simulink model "Plant"  (R2021a)
settings: Solver=VariableStepAuto  StartTime=0.0  StopTime=10.0  RelTol=1e-3
values from neighbouring files (symbols this model uses):
  I = [Jx Jxy Jxz ... (first row only)    [init.m]
  m = 1.5    [init.m]
  pos_ref = [ pos_refx' pos_refy' pos_refz' ]    [trajplann3.m]
  t_ref = []    [trajplann3.m]
  vel_ref = [ vel_refx, vel_refy, vel_refz ]    [trajplann3.m]
undefined symbols (not defined in the file or in its folder): psi, psi_dot
libraries: simulink x2
settings Model: Creator=iris  LastModifiedBy=iris

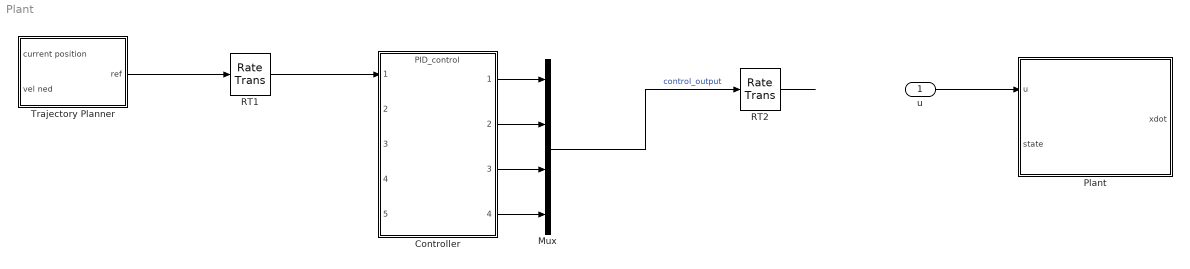
== system Plant ==
  u : Inport
  Controller : ModelReference  ModelNameDialog=PID_control  SimulationMode=Normal  ModelReferenceVersion=4.0
  Mux : Mux
  Plant : Subsystem
  RT1 : RateTransition  OutPortSampleTimeOpt=Inherit  OutPortSampleTime=0.01
  RT2 : RateTransition  OutPortSampleTimeOpt=Inherit  OutPortSampleTime=0.001
  Trajectory Planner : Subsystem
  wires:
  Controller/1 -> Mux/1
  Controller/2 -> Mux/2
  Controller/3 -> Mux/3
  Controller/4 -> Mux/4
  Trajectory Planner/1(ref) -> RT1/1
  RT1/1 -> Controller/1
  u/1 -> Plant/1(u)
  Mux/1 -> RT2/1  "control_output"
  RT2/1 -> ?

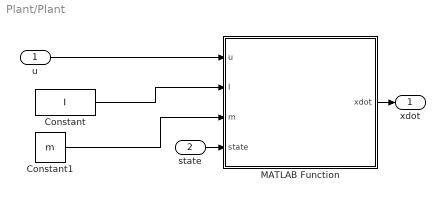
== system Plant/Plant ==
  u : Inport
  state : Inport  Port=2
  Constant : Constant  Value=I
  Constant1 : Constant  Value=m
  MATLAB Function : MATLAB Function  TreatAsAtomicUnit=on
  xdot : Outport
  wires:
  u/1 -> MATLAB Function/1(u)
  Constant1/1 -> MATLAB Function/3(m)
  MATLAB Function/1(xdot) -> xdot/1
  Constant/1 -> MATLAB Function/2(I)
  state/1 -> MATLAB Function/4(state)

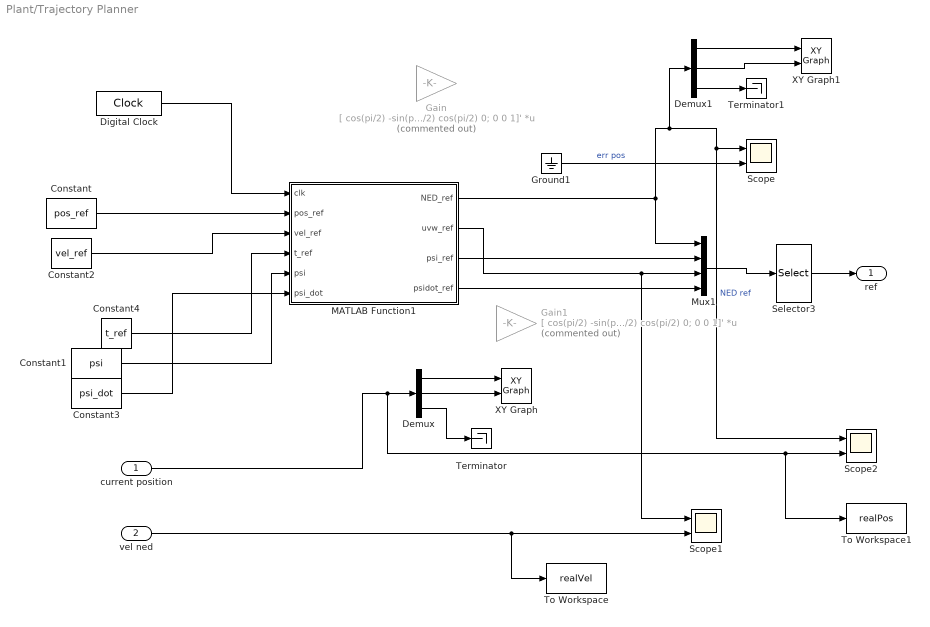
== system Plant/Trajectory Planner ==
  current position : Inport
  vel ned : Inport  Port=2
  Constant : Constant  Value=pos_ref
  Constant1 : Constant  Value=psi
  Constant2 : Constant  Value=vel_ref
  Constant3 : Constant  Value=psi_dot
  Constant4 : Constant  Value=t_ref
  Demux : Demux  Outputs=3
  Demux1 : Demux  Outputs=3
  Digital Clock : DigitalClock  SampleTime=-1
  Gain : Gain  Commented=on  Gain=[ cos(pi/2) -sin(pi/2) 0; -sin(pi/2) cos(pi/2) 0; 0 0 1]'  Multiplication=Matrix(K*u)
  Gain1 : Gain  Commented=on  Gain=[ cos(pi/2) -sin(pi/2) 0; sin(pi/2) cos(pi/2) 0; 0 0 1]'  Multiplication=Matrix(K*u)
  Ground1 : Ground
  MATLAB Function1 : MATLAB Function  TreatAsAtomicUnit=on
  Mux1 : Mux
  Scope : Scope  NumInputPorts=2
  Scope1 : Scope  NumInputPorts=2
  Scope2 : Scope  NumInputPorts=2
  Selector3 : Selector  InputPortWidth=8  IndexOptions=Index vector (dialog)  Indices=[1 5 2 6 4 3 7 8]  OutputSizes=1
  Terminator : Terminator
  Terminator1 : Terminator
  To Workspace : ToWorkspace  VariableName=realVel  SaveFormat=Timeseries  SampleTime=-1
  To Workspace1 : ToWorkspace  VariableName=realPos  SaveFormat=Timeseries  SampleTime=-1
  XY Graph : simulink/Sinks/XY Graph  xmin=-20  xmax=20  ymin=-20  ymax=20  st=-1
  XY Graph1 : simulink/Sinks/XY Graph  xmin=-20  xmax=20  ymin=-20  ymax=20  st=-1
  ref : Outport  VectorParamsAs1DForOutWhenUnconnected=off
  wires:
  MATLAB Function1/3(psi_ref) -> Mux1/2
  Mux1/1 -> Selector3/1
  MATLAB Function1/1(NED_ref) -> Demux1/1, Scope2/1, Scope/1, Mux1/1  "NED ref"
  Selector3/1 -> ref/1
  Constant/1 -> MATLAB Function1/2(pos_ref)
  Constant2/1 -> MATLAB Function1/3(vel_ref)
  current position/1 -> To Workspace1/1, Scope2/2, Demux/1
  Ground1/1 -> Scope/2  "err pos"
  Demux/2 -> XY Graph/2
  Demux/1 -> XY Graph/1
  Demux/3 -> Terminator/1
  Demux1/1 -> XY Graph1/1
  Demux1/2 -> XY Graph1/2
  Demux1/3 -> Terminator1/1
  vel ned/1 -> To Workspace/1, Scope1/2
  Constant4/1 -> MATLAB Function1/4(t_ref)
  Digital Clock/1 -> MATLAB Function1/1(clk)
  MATLAB Function1/2(uvw_ref) -> Scope1/1, Mux1/3
  Constant1/1 -> MATLAB Function1/5(psi)
  Constant3/1 -> MATLAB Function1/6(psi_dot)
  MATLAB Function1/4(psidot_ref) -> Mux1/4

== matlab function Plant/MATLAB Function ==
  data: u input; xdot output; I input; m input; state input
function xdot = plant(u,I,m,state)


T = u(1);
phi = state(4);
th  = state(5);
psi = state(6);
p  = state(10);
q  = state(11);
r  = state(12);

i_1 = (I(2,2)-I(3,3))/I(1,1);
i_2 = 1/I(1,1);
i_3 = (I(3,3)-I(1,1))/I(2,2);
i_4 = 1/I(2,2);
i_5 = (I(1,1)-I(2,2))/I(3,3);
i_6 = 1/I(3,3);


Rot_mat = [cos(th)*cos(psi) sin(phi)*sin(th)*cos(psi)-cos(phi)*sin(psi) cos(phi)*sin(th)*cos(psi)+sin(phi)*sin(psi);
    cos(th)*sin(psi) sin(phi)*sin(th)*sin(psi)+cos(phi)*cos(psi) cos(phi)*sin(th)*sin(psi)-sin(phi)*cos(psi);
    -sin(th) sin(phi)*cos(th) cos(phi)*cos(th)];


f = [Rot_mat'*state(7:9)
     p + (sin(phi)*tan(th))*q - (cos(phi)*tan(th))*r
     cos(phi)*q + sin(phi)*r
     -1*sin(phi)*sec(th)*q + cos(phi)*sec(th)*r
     -1/m*(cos(phi)*sin(th)*cos(psi) + sin(phi)sin(psi))*T
     -1/m*(cos(phi)*sin(th)*sin(psi) - sin(phi)cos(psi))*T
     g - 1/m*(cos(phi)*cos(th))*T
     i_1*q*r
     i_3*r*p
     i_5*p*q];
        

g = zeros(12,6);
g(10,4) = i_2;
g(11,5) = i_4;
g(12,6) = i_6;

xdot = f + g*u;

end

== matlab function Plant/Trajectory Planner/MATLAB Function1 ==
  data: clk input; NED_ref output; pos_ref input; vel_ref input; t_ref input; uvw_ref output; psi_ref output; psi input; psi_dot input; psidot_ref output
function [ NED_ref, uvw_ref, psi_ref,psidot_ref] = trajectoryPlanner(clk,pos_ref,vel_ref,t_ref,psi,psi_dot)

currTime = find(clk >= t_ref);
NED_ref = pos_ref(currTime(end),:)';
uvw_ref = vel_ref(currTime(end),:)';
psi_ref = psi(currTime(end),:)';
psidot_ref = psi_dot(currTime(end),:)';

end
